simulink model "p4"  (R2020a)
settings: Solver=ode15s  StartTime=0.0  StopTime=0.2  RelTol=1e-3
model workspace (MAT data in the model file):
  B = 3.5077e-06
  J = 3.2284e-06
  K = 0.0274
  Kd = 0.15
  Ki = 500
  Kp = 21
  L = 2.75e-06
  R = 4
settings Model: DataDictionary=prob4_data.sldd  OrderedModelArguments=off  Creator=007  LastModifiedBy=007

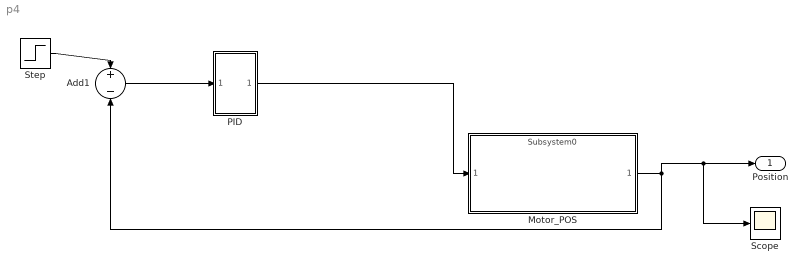
== system p4 ==
  Add1 : Sum  Inputs=+-
  Motor_POS : ModelReference  ModelNameDialog=Subsystem0  ModelReferenceVersion=1.7
  PID : Subsystem
  Scope : Scope
  Step : Step  Time=0  SampleTime=0
  Position : Outport
  wires:
  Step/1 -> Add1/1
  Motor_POS/1 -> Scope/1, Position/1, Add1/2
  Add1/1 -> PID/1(Input)
  PID/1(Output) -> Motor_POS/1

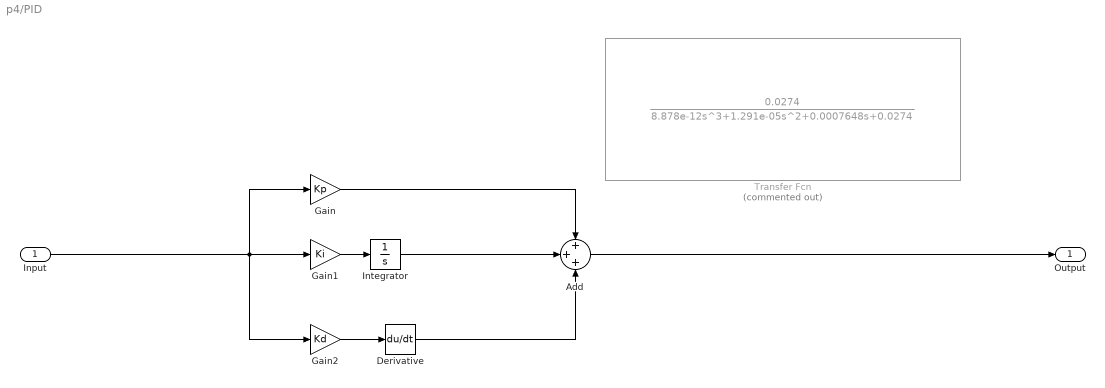
== system p4/PID ==
  Input : Inport
  Add : Sum  Inputs=+++
  Derivative : Derivative
  Gain : Gain  Gain=Kp
  Gain1 : Gain  Gain=Ki
  Gain2 : Gain  Gain=Kd
  Integrator : Integrator
  Transfer Fcn : TransferFcn  Commented=on  Numerator=[0.0274]  Denominator=[8.878e-12 1.291e-05 0.0007648 0.0274]
  Output : Outport
  wires:
  Gain/1 -> Add/1
  Gain2/1 -> Derivative/1
  Derivative/1 -> Add/3
  Gain1/1 -> Integrator/1
  Integrator/1 -> Add/2
  Input/1 -> Gain2/1, Gain/1, Gain1/1
  Add/1 -> Output/1
